simulink model "Driveline_ctrl_sim"  (R2020a)
settings: Solver=ode45  StartTime=0.0  StopTime=50  MaxStep=0.001  RelTol=1e-3
values from neighbouring files (symbols this model uses):
  A = [[-1/tau 0];[1/m -rho*CD*Af*x2e/m]]    [CruiseCtrl_StateFeedback_Int_design.m]
  B = [k*r/tau/rw 0]'    [CruiseCtrl_StateFeedback_Int_design.m]
  C = [0 1]    [CruiseCtrl_StateFeedback_Int_design.m]
  D = [0]    [CruiseCtrl_StateFeedback_Int_design.m]
undefined symbols (not defined in the file or in its folder): G, K, kr, M, phi, R, x0
libraries: simulink_extras x1
settings Model: Creator=jofr  LastModifiedBy=juan
settings DataIOCC: LimitDataPoints=on  SaveFormat=Array  SignalLoggingSaveFormat=ModelDataLogs  ReturnWorkspaceOutputs=off
settings OptimizationCC: BlockReduction=off  BooleanDataType=off  LifeSpan=inf
settings DebuggingCC: SaveWithParameterizedLinksMsg=none  UnderspecifiedInitializationDetection=Classic  MergeDetectMultiDrivingBlocksExec=none  SignalResolutionControl=TryResolveAllWithWarning  MultiTaskDSMMsg=warning  MultiTaskCondExecSysMsg=none  SFUnexpectedBacktrackingDiag=warning  SFNoUnconditionalDefaultTransitionDiag=warning  SFExecutionAtInitializationDiag=none  ArithmeticOperatorsInVariantConditions=warning
settings HardwareCC: ProdBitPerPointer=32  ProdBitPerSizeT=32  ProdBitPerPtrDiffT=32  ProdLargestAtomicFloat=None  ProdIntDivRoundTo=Undefined  ProdEndianess=Unspecified  ProdWordSize=32  ProdHWDeviceType=32-bit Generic  TargetUnknown=on
settings ModelReferenceCC: PropagateSignalLabelsOutOfModel=off
settings SFSimCC: SimUseLocalCustomCode=off  CustomCodeUndefinedFunction=UseInterfaceOnly
settings RTWCC: RTWUseLocalCustomCode=off
settings CodeAppCC: StateflowObjectComments=on
settings GRTTargetCC: TargetLangStandard=C89/C90 (ANSI)
settings ConfigComp: CovMetricSettings=dw  CovHtmlReporting=on  CovSaveCumulativeToWorkspaceVar=on  CovSaveSingleToWorkspaceVar=on  CovExternalEMLEnable=off

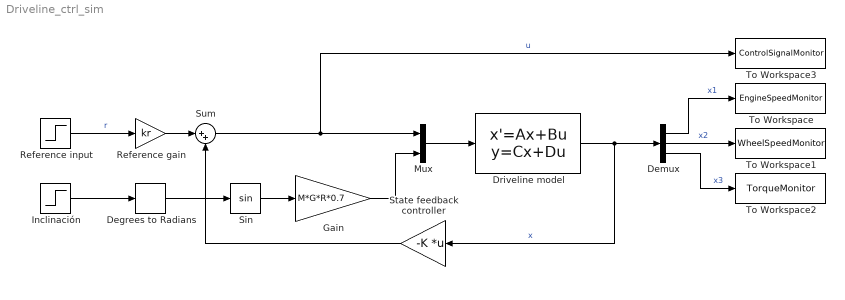
== system Driveline_ctrl_sim ==
  Degrees to Radians : simulink_extras/Transformations/Degrees to Radians
  Demux : Demux  Outputs=3
  Driveline model : StateSpace  A=A  B=B  C=C  D=D  InitialCondition=x0
  Gain : Gain  Gain=M*G*R*0.7
  Inclinación : Step  Time=10  After=phi  SampleTime=0
  Mux : Mux  Inputs=2
  Reference gain : Gain  Gain=kr
  Reference input : Step  Before=2  After=4  SampleTime=0
  Sin : Trigonometry
  State feedback controller : Gain  Gain=-K  Multiplication=Matrix(K*u)
  Sum : Sum  Inputs=|++
  To Workspace : ToWorkspace  VariableName=EngineSpeedMonitor  SaveFormat=Structure With Time  SampleTime=-1
  To Workspace1 : ToWorkspace  VariableName=WheelSpeedMonitor  SaveFormat=Structure With Time  SampleTime=-1
  To Workspace2 : ToWorkspace  VariableName=TorqueMonitor  SaveFormat=Structure With Time  SampleTime=-1
  To Workspace3 : ToWorkspace  VariableName=ControlSignalMonitor  SaveFormat=Structure With Time  SampleTime=-1
  wires:
  Driveline model/1 -> State feedback controller/1, Demux/1  "x"
  Demux/1 -> To Workspace/1  "x1"
  Mux/1 -> Driveline model/1
  State feedback controller/1 -> Sum/2
  Reference input/1 -> Reference gain/1  "r"
  Sum/1 -> To Workspace3/1, Mux/1  "u"
  Reference gain/1 -> Sum/1
  Demux/2 -> To Workspace1/1  "x2"
  Demux/3 -> To Workspace2/1  "x3"
  Inclinación/1 -> Degrees to Radians/1
  Degrees to Radians/1 -> Sin/1
  Sin/1 -> Gain/1
  Gain/1 -> Mux/2
